simulink model "rgb2gray_fpga"  (R2013a)
settings: Solver=ode45  StartTime=0.0  StopTime=348*512*3  RelTol=1e-3
undefined symbols (not defined in the file or in its folder): gray
libraries: xbsIndex_r4 x14, dspmtrx3 x4, visionsinks x2, visionsources x1, dspsigattribs x1
settings Model: Creator=diegohr  LastModifiedBy=diego

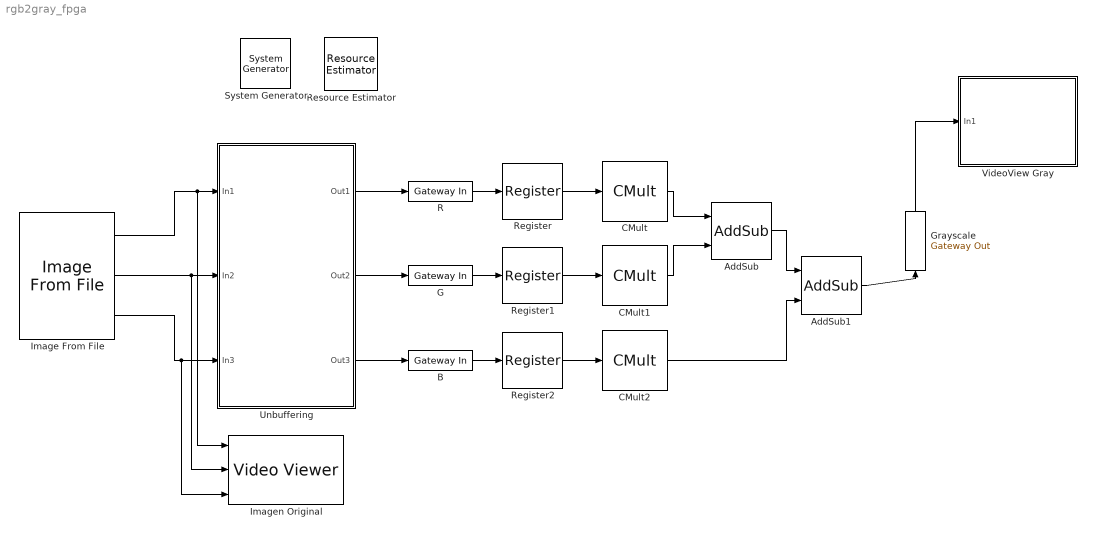
== system rgb2gray_fpga ==
  " System Generator" : xbsIndex_r4/ System Generator  Tag=genX  xilinxfamily=spartan6  part=xc6slx45t  speed=-3  package=fgg484  synthesis_tool=XST  clock_wrapper=Clock Enables  directory=./netlist  proj_type=Project Navigator  Synth_file=XST Defaults  Impl_file=ISE Defaults  testbench=off  simulink_period=5.0863e-06  sysclk_period=15  dcm_input_clock_period=10  incr_netlist=off  trim_vbits=Everywhere in SubSystem  dbl_ovrd=According to Block Masks  core_generation=According to Block Masks  run_coregen=off  deprecated_control=off  eval_field=0  block_type=sysgen
  AddSub : xbsIndex_r4/AddSub  mode=Addition  use_carryin=off  use_carryout=off  en=off  latency=0  precision=Full  arith_type=Unsigned  n_bits=16  bin_pt=14  quantization=Truncate  overflow=Wrap  dbl_ovrd=off  use_behavioral_HDL=off  hw_selection=Fabric  pipelined=off  block_type=addsub
  AddSub1 : xbsIndex_r4/AddSub  mode=Addition  use_carryin=off  use_carryout=off  en=off  latency=0  precision=Full  arith_type=Unsigned  n_bits=16  bin_pt=14  quantization=Truncate  overflow=Wrap  dbl_ovrd=off  use_behavioral_HDL=off  hw_selection=Fabric  pipelined=off  block_type=addsub
  B : xbsIndex_r4/Gateway In  gui_display_data_type=Fixed-point  arith_type=Unsigned  n_bits=16  bin_pt=14  preci_type=Single  exp_width=8  frac_width=24  quantization="Round  (unbiased: +/- Inf)"  overflow=Saturate  period=5.0863e-06  dbl_ovrd=off  timing_constraint=None  locs_specified=off  LOCs={}  UseAsADC=off  ADCChannel='1'  inherit_from_input=off  hdl_port=on  block_type=gatewayin
  CMult : xbsIndex_r4/CMult  const=0.2989  gui_display_data_type=Fixed-point  const_n_bits=16  const_bin_pt=14  float_type=Single  exp_bits=8  fraction_bits=24  en=off  latency=0  precision=Full  arith_type="Signed  (2's comp)"  n_bits=16  bin_pt=14  quantization=Truncate  overflow=Wrap  dbl_ovrd=off  use_behavioral_HDL=off  mem_type=Distributed RAM  pipeline=off  block_type=cmult
  CMult1 : xbsIndex_r4/CMult  const=0.5870  gui_display_data_type=Fixed-point  const_n_bits=16  const_bin_pt=14  float_type=Single  exp_bits=8  fraction_bits=24  en=off  latency=0  precision=Full  arith_type="Signed  (2's comp)"  n_bits=16  bin_pt=14  quantization=Truncate  overflow=Wrap  dbl_ovrd=off  use_behavioral_HDL=off  mem_type=Distributed RAM  pipeline=off  block_type=cmult
  CMult2 : xbsIndex_r4/CMult  const=0.1140  gui_display_data_type=Fixed-point  const_n_bits=16  const_bin_pt=14  float_type=Single  exp_bits=8  fraction_bits=24  en=off  latency=0  precision=Full  arith_type="Signed  (2's comp)"  n_bits=16  bin_pt=14  quantization=Truncate  overflow=Wrap  dbl_ovrd=off  use_behavioral_HDL=off  mem_type=Distributed RAM  pipeline=off  block_type=cmult
  G : xbsIndex_r4/Gateway In  gui_display_data_type=Fixed-point  arith_type=Unsigned  n_bits=16  bin_pt=14  preci_type=Single  exp_width=8  frac_width=24  quantization="Round  (unbiased: +/- Inf)"  overflow=Saturate  period=5.0863e-06  dbl_ovrd=off  timing_constraint=None  locs_specified=off  LOCs={}  UseAsADC=off  ADCChannel='1'  inherit_from_input=off  hdl_port=on  block_type=gatewayin
  Grayscale : xbsIndex_r4/Gateway Out  inherit_from_input=off  hdl_port=off  timing_constraint=None  locs_specified=off  LOCs={}  UseAsDAC=off  DACChannel='1'  block_type=gatewayout
  Image From File : visionsources/Image From File  Tag=vipblks_nd  FileName=peppers.png  imagePorts=Separate color signals  Ts=inf  ImageDataType=double  Signed=on  WordLength=16  sdImageDataType=uint(8)  FractionLengthMode=User-defined  FractionLength=15  OutPortLabels=R|G|B
  Imagen Original : visionsinks/Video Viewer  inputType=Obsolete7b  imagePorts=Separate color signals  useColorMap=off  colormapValue=gray(256)  specRange=off  minInputVal=0  maxInputVal=255  FigPos=[263 777 739 516]  AxisZoom=on  trueSizedOnce=off  OpenAtMdlStart=on  DefaultConfigurationName=vipscopes.VideoViewerScopeCfg
  R : xbsIndex_r4/Gateway In  gui_display_data_type=Fixed-point  arith_type=Unsigned  n_bits=16  bin_pt=14  preci_type=Single  exp_width=8  frac_width=24  quantization="Round  (unbiased: +/- Inf)"  overflow=Saturate  period=5.0863e-06  dbl_ovrd=off  timing_constraint=None  locs_specified=off  LOCs={}  UseAsADC=off  ADCChannel='1'  inherit_from_input=off  hdl_port=on  block_type=gatewayin
  Register : xbsIndex_r4/Register  init=0  rst=off  en=off  dbl_ovrd=off  block_type=register
  Register1 : xbsIndex_r4/Register  init=0  rst=off  en=off  dbl_ovrd=off  block_type=register
  Register2 : xbsIndex_r4/Register  init=0  rst=off  en=off  dbl_ovrd=off  block_type=register
  Resource Estimator : xbsIndex_r4/Resource Estimator  Tag=resEstTag  Slices=0  FFs=0  BRAMs=0  LUTs=0  IOBs=0  EBMs=0  TBUFs=0  xl_use_estimator_area=off  est_options=Post Map  block_type=resource_estimator
      settings: AttributesFormatString=Resource\nEstimator
  Unbuffering : Subsystem
  VideoView Gray : Subsystem
  wires:
  Image From File/2 -> Imagen Original/2, Unbuffering/2(In2)
  Image From File/1 -> Imagen Original/1, Unbuffering/1(In1)
  Image From File/3 -> Imagen Original/3, Unbuffering/3(In3)
  Unbuffering/2(Out2) -> G/1
  Unbuffering/1(Out1) -> R/1
  Unbuffering/3(Out3) -> B/1
  R/1 -> Register/1
  G/1 -> Register1/1
  B/1 -> Register2/1
  Register/1 -> CMult/1
  Register1/1 -> CMult1/1
  Register2/1 -> CMult2/1
  CMult/1 -> AddSub/1
  CMult1/1 -> AddSub/2
  CMult2/1 -> AddSub1/2
  AddSub/1 -> AddSub1/1
  AddSub1/1 -> Grayscale/1
  Grayscale/1 -> VideoView Gray/1(In1)

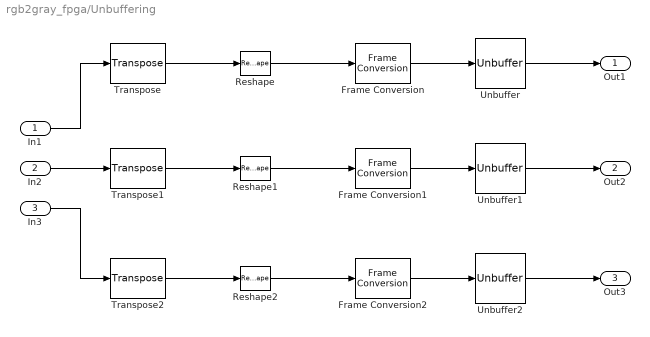
== system rgb2gray_fpga/Unbuffering ==
  In1 : Inport
  In2 : Inport  Port=2
  In3 : Inport  Port=3
  Frame Conversion : FrameConversion
  Frame Conversion1 : FrameConversion
  Frame Conversion2 : FrameConversion
  Reshape : Reshape
  Reshape1 : Reshape
  Reshape2 : Reshape
  Transpose : dspmtrx3/Transpose  Hermitian=off  overflowFlag=off
  Transpose1 : dspmtrx3/Transpose  Hermitian=off  overflowFlag=off
  Transpose2 : dspmtrx3/Transpose  Hermitian=off  overflowFlag=off
  Unbuffer : Unbuffer  SampleBasedProcessing=Same as frame based
  Unbuffer1 : Unbuffer  SampleBasedProcessing=Same as frame based
  Unbuffer2 : Unbuffer  SampleBasedProcessing=Same as frame based
  Out1 : Outport
  Out2 : Outport  Port=2
  Out3 : Outport  Port=3
  wires:
  In1/1 -> Transpose/1
  In3/1 -> Transpose2/1
  Reshape2/1 -> Frame Conversion2/1
  Frame Conversion1/1 -> Unbuffer1/1
  Transpose/1 -> Reshape/1
  Unbuffer/1 -> Out1/1
  Reshape1/1 -> Frame Conversion1/1
  Transpose2/1 -> Reshape2/1
  Reshape/1 -> Frame Conversion/1
  Unbuffer1/1 -> Out2/1
  Unbuffer2/1 -> Out3/1
  Frame Conversion/1 -> Unbuffer/1
  Frame Conversion2/1 -> Unbuffer2/1
  In2/1 -> Transpose1/1
  Transpose1/1 -> Reshape1/1

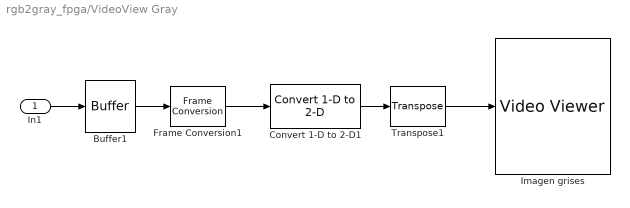
== system rgb2gray_fpga/VideoView Gray ==
  In1 : Inport
  Buffer1 : Buffer  N=196608  TreatMby1Signals=One channel
  Convert 1-D to 2-D1 : dspsigattribs/Convert 1-D to 2-D  M=512  N=384  frameBasedOut=off
  Frame Conversion1 : FrameConversion
  Imagen grises : visionsinks/Video Viewer  inputType=Obsolete7b  imagePorts=One multidimensional signal  useColorMap=off  colormapValue=gray(256)  specRange=off  minInputVal=0  maxInputVal=255  FigPos=[1005 774 742 513]  AxisZoom=on  trueSizedOnce=off  OpenAtMdlStart=on  DefaultConfigurationName=vipscopes.VideoViewerScopeCfg
  Transpose1 : dspmtrx3/Transpose  Hermitian=off  overflowFlag=off
  wires:
  Convert 1-D to 2-D1/1 -> Transpose1/1
  Buffer1/1 -> Frame Conversion1/1
  Frame Conversion1/1 -> Convert 1-D to 2-D1/1
  Transpose1/1 -> Imagen grises/1
  In1/1 -> Buffer1/1
